simulink model "PlantaPIL"  (R2022b)
settings: Solver=ode1  StartTime=0.0  StopTime=SIMULPARAM.T_end  FixedStep=SIMULPARAM.Ts  RelTol=1e-3  EnableMultiTasking=on
InitFcn:
  | System_Parameters;
StopFcn:
  | ShowResults;
undefined symbols (not defined in the file or in its folder): Bat_cell, C_fil, C_fil_0, ENV, IPM, Ki_current_bat, Ki_current_sc, Ki_d_cur, Ki_q_cur, Kp_current_bat, Kp_current_sc, Kp_d_cur, Kp_q_cur, Kp_voltage, Kp_Vveh, L_bat, L_sc, n_bat_par, n_bat_seri, n_sc_par, n_sc_seri, Nbat, Ninv, Nsc, P1_I, P_I, R1_on, R_on, Rth, SC_modul, SC_pack, u_dc_ref, VEH
libraries: esp32_device_config_lib x1, simulink x1
(part 1 of 2)
settings Model: DataDictionary=MySharedDict.sldd  SILPILSystemUnderTest=refmodels  CodeVerificationMode=processor-in-the-loop (pil)  Creator=coins  LastModifiedBy=crist
settings SolverCC: AlgebraicLoopSolver=LineSearch  PositivePriorityOrder=on  AutoInsertRateTranBlk=on
settings DataIOCC: SignalLogging=off
settings OptimizationCC: EnhancedBackFolding=on  PassReuseOutputArgsAs=Individual arguments  ZeroExternalMemoryAtStartup=off  ZeroInternalMemoryAtStartup=off  OptimizeBlockOrder=speed  DifferentSizesBufferReuse=on  OptimizationCustomize=off  EfficientTunableParamExpr=on
settings DebuggingCC: ParameterTunabilityLossMsg=error  UnconnectedInputMsg=warning  UnconnectedOutputMsg=warning  UnconnectedLineMsg=warning  ModelReferenceSymbolNameMessage=none  PregeneratedLibrarySubsystemCodeDiagnostic=none  SFMachineParentedDataDiag=warning  ArithmeticOperatorsInVariantConditions=warning
settings HardwareCC: ProdBitPerPointer=32  ProdBitPerSizeT=32  ProdBitPerPtrDiffT=32  ProdLargestAtomicInteger=Long  ProdLargestAtomicFloat=Double  ProdWordSize=32  ProdHWDeviceType=Cadence Design Systems (Tensilica)->Espressif Xtensa single-/dual-core 32-bit LX6 microprocessor
settings ModelReferenceCC: UpdateModelReferenceTargets=Force  EnableRefExpFcnMdlSchedulingChecks=on
settings SFSimCC: MATLABDynamicMemAlloc=off  CustomCodeUndefinedFunction=UseInterfaceOnly
settings RTWCC: Description=Waijung 2 ESP32 target  SystemTargetFile=esp32.tlc  TemplateMakefile=esp32.tmf  RetainRTWFile=on  CreateSILPILBlock=PIL  CodeExecutionProfiling=on  DLArmComputeVersion=19.05
settings CodeAppCC: ForceParamTrailComments=on  IgnoreCustomStorageClasses=off  OperatorAnnotations=on  SimulinkDataObjDesc=on  SFDataObjDesc=on  InsertBlockDesc=on
settings STFCustomTargetCC: TargetLangStandard=C99 (ISO)  MultiwordLength=256  ModelReferenceCompliant=off  CombineOutputUpdateFcns=on  ERTCustomFileBanners=on  SupportContinuousTime=off  SupportNonInlinedSFcns=off  RemoveResetFunc=on  MATLABClassNameForMDSCustomization=Simulink.SoftwareTarget.ERTCustomization  SystemTargetFile=esp32.tlc
settings ERTTargetCC: TargetLangStandard=C99 (ISO)  ModelReferenceCompliant=off  ParMdlRefBuildCompliant=off  CompOptLevelCompliant=off  ConcurrentExecutionCompliant=off  ModelStepFunctionPrototypeControlCompliant=off  CPPClassGenCompliant=off  UseToolchainInfoCompliant=off  ExtModeStaticAlloc=on  ExtModeStaticAllocSize=2048  ERTSrcFileBannerTemplate=esp32_code_template.cgt  ERTHdrFileBannerTemplate=esp32_code_template.cgt  ERTDataSrcFileTemplate=esp32_code_template.cgt  ERTDataHdrFileTemplate=esp32_code_template.cgt  ERTCustomFileTemplate=esp32_file_process.tlc

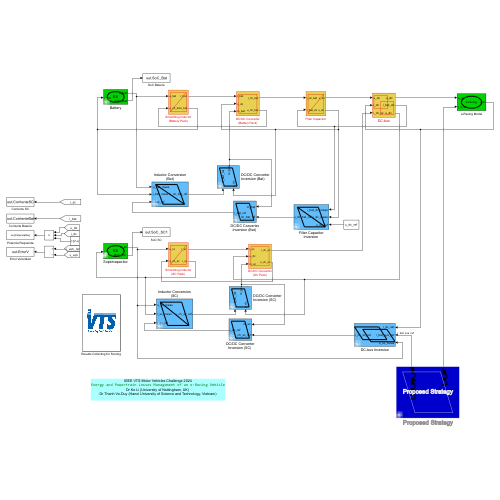
[thumbnail: Simulink's stored preview of the top-level diagram]
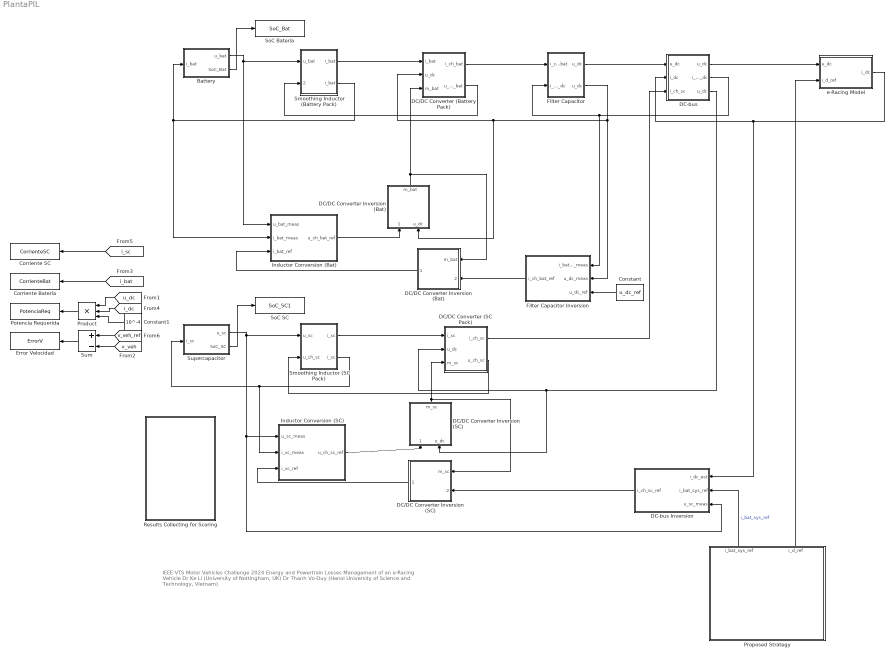
== system PlantaPIL ==
  note: IEEE VTS Motor Vehicles Challenge 2024
      | Energy and Powertrain Losses Management of an e-Racing Vehicle
      | Dr Ke Li (University of Nottingham, UK)
      | Dr Thanh Vo-Duy (Hanoi University of Science and Technology, Vietnam)
  Battery : Subsystem  AncestorBlock=simulink/REM/SE
      mask Display:
      | plot(0,0,100,100, 1.2*[50,57.68,60.77,63.08,64.97,66.58,68,69.26,70.4, 	71.42,72.36,78.28,80,78.28,72.36,71.42,70.4, 	69.26,68,66.58,64.97,63.08,60.77,57.68,50,42.32, 	39.23,36.92,35.03,33.42,32,30.74,29.6,28.58, 	27.64,21.72,20,21.72,27.64,28.58,29.6,30.74,32, 	33.42,35.03,36.92,39.23,42.32,50]-10, 1.2*[20,21,22,23,24,25,26,27,28,29,30,40,50,60,70,71,72, 	73,74,75,76,77,78,79,80,79,78,77,76,75,74,73,72, 	71,70,60,50,40,30,29,28,27,26,25,24,23,22,21,20]-10)
      | disp('ES')
  Constant : Constant  Value=u_dc_ref
  Constant1 : Constant  Value=10^-4
  Corriente Batería : ToWorkspace  VariableName=CorrienteBat  SaveFormat=Structure With Time  SampleTime=-1
  Corriente SC : ToWorkspace  VariableName=CorrienteSC  SaveFormat=Structure With Time  SampleTime=-1
  DC-bus : Subsystem  mask(CM){}
      mask Display: plot(0,0,100,100,[35,35,95,95,35],[65,10,10,65,65], [5,5,65,65,5],[90,35,35,90,90])
  DC-bus Inversion : Subsystem  AncestorBlock=simulink/SMC/Bloc de pondération
      mask Display: plot(0,0,100,100,[20,40,100,80,20],[75,20,20,75,75], [0,20,80,60,0],[85,30,30,85,85])
  DC/DC Converter (Battery Pack) : Subsystem
      mask Display: plot(0,0,100,100,[10,10,90,90,10],[90,10,10,90,90])
  DC/DC Converter (SC Pack) : Subsystem
      mask Display: plot(0,0,100,100,[10,10,90,90,10],[90,10,10,90,90])
  "DC/DC Converter Inversion (Bat) " : Subsystem  AncestorBlock=simulink/SMC/Inversion EC avec mesure
      mask Display: plot(0,0,100,100,[10,30,90,70,10],[90,10,10,90,90])
  "DC/DC Converter Inversion (Bat)  " : Subsystem  AncestorBlock=simulink/SMC/Inversion EC avec mesure
      mask Display: plot(0,0,100,100,[10,30,90,70,10],[90,10,10,90,90])
  DC/DC Converter Inversion (SC) : Subsystem  AncestorBlock=simulink/SMC/Inversion EC avec mesure
      mask Display: plot(0,0,100,100,[10,30,90,70,10],[90,10,10,90,90])
  "DC/DC Converter Inversion (SC) " : Subsystem  AncestorBlock=simulink/SMC/Inversion EC avec mesure
      mask Display: plot(0,0,100,100,[10,30,90,70,10],[90,10,10,90,90])
  Error Velocidad : ToWorkspace  VariableName=ErrorV  SaveFormat=Structure With Time  SampleTime=-1
  Filter Capacitor : Subsystem  mask(CM){}
      mask Display: plot(0,0,100,100,[10,10,90,90,10],[90,10,10,90,90], [10,90],[10,90])
  "Filter Capacitor Inversion " : Subsystem  AncestorBlock=simulink/SMC/Asservissement Correcteur IP
      mask Display: plot(0,0,100,100, [10,30,90,70,10,90],[90,10,10,90,90,10])
  Inductor Conversion (Bat) : Subsystem  AncestorBlock=simulink/SMC/Asservissement Correcteur IP
      mask Display: plot(0,0,100,100, [10,30,90,70,10,90],[90,10,10,90,90,10])
  Inductor Conversion (SC) : Subsystem  AncestorBlock=simulink/SMC/Asservissement Correcteur IP
      mask Display: plot(0,0,100,100, [10,30,90,70,10,90],[90,10,10,90,90,10])
  Potencia Requerida : ToWorkspace  VariableName=PotenciaReq  SaveFormat=Structure With Time  SampleTime=-1
  Product : Product  Inputs=3
  Proposed Strategy : Subsystem  AncestorBlock=simulink/SMC/Inversion EC avec mesure
      mask Display:
      | disp('Proposed Strategy')
      | plot(0,0,100,100,[10,30,90,70,10],[90,10,10,90,90])
  Results Collecting for Scoring : Subsystem
      mask Display: image('VTS.png');
  Smoothing Inductor (Battery Pack) : Subsystem  mask(CM){}
      mask Display: plot(0,0,100,100,[10,10,90,90,10],[90,10,10,90,90], [10,90],[10,90])
  Smoothing Inductor (SC Pack) : Subsystem  mask(CM){}
      mask Display: plot(0,0,100,100,[10,10,90,90,10],[90,10,10,90,90], [10,90],[10,90])
  SoC Batería : ToWorkspace  VariableName=SoC_Bat  SaveFormat=Structure With Time  SampleTime=-1
  SoC SC : ToWorkspace  VariableName=SoC_SC1  SaveFormat=Structure With Time  SampleTime=-1
  Sum : Sum  Inputs=+-
  Supercapacitor : Subsystem  AncestorBlock=simulink/REM/SE
      mask Display:
      | plot(0,0,100,100, 1.2*[50,57.68,60.77,63.08,64.97,66.58,68,69.26,70.4, 	71.42,72.36,78.28,80,78.28,72.36,71.42,70.4, 	69.26,68,66.58,64.97,63.08,60.77,57.68,50,42.32, 	39.23,36.92,35.03,33.42,32,30.74,29.6,28.58, 	27.64,21.72,20,21.72,27.64,28.58,29.6,30.74,32, 	33.42,35.03,36.92,39.23,42.32,50]-10, 1.2*[20,21,22,23,24,25,26,27,28,29,30,40,50,60,70,71,72, 	73,74,75,76,77,78,79,80,79,78,77,76,75,74,73,72, 	71,70,60,50,40,30,29,28,27,26,25,24,23,22,21,20]-10)
      | disp('ES')
  e-Racing Model : Subsystem
      mask Display:
      | plot(0,0,100,100, 1.2*[50,57.68,60.77,63.08,64.97,66.58,68,69.26,70.4, 	71.42,72.36,78.28,80,78.28,72.36,71.42,70.4, 	69.26,68,66.58,64.97,63.08,60.77,57.68,50,42.32, 	39.23,36.92,35.03,33.42,32,30.74,29.6,28.58, 	27.64,21.72,20,21.72,27.64,28.58,29.6,30.74,32, 	33.42,35.03,36.92,39.23,42.32,50]-10, 1.2*[20,21,22,23,24,25,26,27,28,29,30,40,50,60,70,71,72, 	73,74,75,76,77,78,79,80,79,78,77,76,75,74,73,72, 	71,70,60,50,40,30,29,28,27,26,25,24,23,22,21,20]-10)
      | disp('e-racing')
  wires:
  Supercapacitor/1(u_sc) -> DC-bus Inversion/3(u_sc_meas), Inductor Conversion (SC)/1(u_sc_meas), Smoothing Inductor (SC Pack)/1(u_sc)
  Smoothing Inductor (SC Pack)/2(i_sc) -> Supercapacitor/1(i_sc), Inductor Conversion (SC)/2(i_sc_meas)
  Smoothing Inductor (SC Pack)/1("i_sc ") -> DC/DC Converter (SC Pack)/1(i_sc)
  DC/DC Converter (SC Pack)/2(u_ch_sc) -> Smoothing Inductor (SC Pack)/2(u_ch_sc)
  DC-bus/1("u_dc  ") -> e-Racing Model/1(u_dc)
  DC/DC Converter (SC Pack)/1(i_ch_sc) -> DC-bus/3(i_ch_sc)
  DC-bus/3("u_dc   ") -> DC/DC Converter Inversion (SC)/2(u_dc), DC/DC Converter (SC Pack)/2(u_dc)
  Battery/1(u_bat) -> Inductor Conversion (Bat)/1(u_bat_meas), Smoothing Inductor (Battery Pack)/1(u_bat)
  Smoothing Inductor (Battery Pack)/2(i_bat) -> Inductor Conversion (Bat)/2(i_bat_meas), Battery/1(i_bat)
  Filter Capacitor/2("u_dc ") -> DC/DC Converter (Battery Pack)/2(u_dc), "DC/DC Converter Inversion (Bat)  "/2(u_dc), "Filter Capacitor Inversion "/2(u_dc_meas)
  Constant/1 -> "Filter Capacitor Inversion "/3(u_dc_ref)
  "DC/DC Converter Inversion (Bat)  "/1(m_bat) -> DC/DC Converter (Battery Pack)/3(m_bat), "DC/DC Converter Inversion (Bat) "/1(m_bat)
  "DC/DC Converter Inversion (SC) "/1(i_sc_ref) -> Inductor Conversion (SC)/3(i_sc_ref)
  Inductor Conversion (SC)/1(u_ch_sc_ref) -> DC/DC Converter Inversion (SC)/1(u_ch_sc_ref)
  DC/DC Converter Inversion (SC)/1(m_sc) -> DC/DC Converter (SC Pack)/3(m_sc), "DC/DC Converter Inversion (SC) "/1(m_sc)
  "Filter Capacitor Inversion "/1(i_ch_bat_ref) -> "DC/DC Converter Inversion (Bat) "/2(i_ch_bat_ref)
  "DC/DC Converter Inversion (Bat) "/1(i_bat_ref) -> Inductor Conversion (Bat)/3(i_bat_ref)
  Inductor Conversion (Bat)/1(u_ch_bat_ref) -> "DC/DC Converter Inversion (Bat)  "/1(u_ch_bat_ref)
  DC/DC Converter (Battery Pack)/2(u_ch_bat) -> Smoothing Inductor (Battery Pack)/2(u_ch_bat)
  DC/DC Converter (Battery Pack)/1(i_ch_bat) -> Filter Capacitor/1(i_ch_bat)
  Smoothing Inductor (Battery Pack)/1("i_bat ") -> DC/DC Converter (Battery Pack)/1(i_bat)
  e-Racing Model/1(i_dc) -> DC-bus Inversion/1(i_dc_est), DC-bus/2(i_dc)
  Filter Capacitor/1(u_dc) -> DC-bus/1(u_dc)
  DC-bus Inversion/1(i_ch_sc_ref) -> "DC/DC Converter Inversion (SC) "/2(i_ch_sc_ref)
  Proposed Strategy/1(i_bat_sys_ref) -> DC-bus Inversion/2(i_bat_sys_ref)  "i_bat_sys_ref"
  DC-bus/2(i_bat_dc) -> "Filter Capacitor Inversion "/1(i_bat_dc_meas), Filter Capacitor/2(i_bat_dc)
  Proposed Strategy/2("i_d_ref ") -> e-Racing Model/2(i_d_ref)
  Supercapacitor/2("SoC_SC ") -> SoC SC/1
  Battery/2(SoC_Bat) -> SoC Batería/1
  [i_sc] -> Corriente SC/1
  [i_bat] -> Corriente Batería/1
  Constant1/1 -> Product/3
  Product/1 -> Potencia Requerida/1
  [i_dc] -> Product/2
  [u_dc] -> Product/1
  [v_veh] -> Sum/2
  [v_veh_ref] -> Sum/1
  Sum/1 -> Error Velocidad/1

== system PlantaPIL/Battery ==
  i_bat : Inport
  Constant : Constant
  Gain : Gain  Gain=1/(3600*Bat_cell.Capacity)
  Gain1 : Gain  Gain=1/n_bat_par
  Gain2 : Gain  Gain=Bat_cell.InternalRes
  Gain3 : Gain  Gain=n_bat_seri
  Gain4 : Gain  Gain=100
  Gain5 : Gain  Gain=-1
  Integrator : Integrator  InitialCondition=1
  OCV(SoC) : Lookup_n-D  NumberOfTableDimensions=1  BreakpointsForDimension1=Bat_cell.SoC  Table=Bat_cell.OCV  InternalRulePriority=Speed  RndMeth=Simplest
  Subtract : Sum  Inputs=+-
  Subtract1 : Sum  Inputs=+-
  u_bat : Outport  InitialOutput=0  VectorParamsAs1DForOutWhenUnconnected=off
  SoC_Bat : Outport  Port=2  InitialOutput=0  VectorParamsAs1DForOutWhenUnconnected=off
  tag scope: Bat_soc=global, i_bat=global, i_bat_cell=global, u_bat=global, u_bat_cell=global
  wires:
  Gain/1 -> Integrator/1
  i_bat/1 -> [i_bat], Gain1/1
  Gain1/1 -> Gain2/1, Gain5/1, [i_bat_cell]  "i_bat_cell"
  OCV(SoC)/1 -> Subtract1/1  "OCV"
  Gain2/1 -> Subtract1/2
  Subtract1/1 -> [u_bat_cell], Gain3/1  "u_bat_cell"
  Gain3/1 -> [u_bat], u_bat/1
  Constant/1 -> Subtract/1
  Integrator/1 -> Gain4/1, Subtract/2
  Gain4/1 -> SoC_Bat/1, [Bat_soc]  "Battery's SoC"
  Subtract/1 -> OCV(SoC)/1
  Gain5/1 -> Gain/1

== system PlantaPIL/DC-bus ==
  u_dc : Inport
  i_dc : Inport  Port=2
  i_ch_sc : Inport  Port=3
  For scoring : ToWorkspace  VariableName=i_dc_meas  SampleTime=-1
      settings: Decimation=SIMULPARAM.Decimation
  Subtract : Sum  Inputs=+-
  "u_dc  " : Outport  InitialOutput=0  VectorParamsAs1DForOutWhenUnconnected=off
  i_bat_dc : Outport  Port=2  InitialOutput=0  VectorParamsAs1DForOutWhenUnconnected=off
  "u_dc   " : Outport  Port=3  InitialOutput=0  VectorParamsAs1DForOutWhenUnconnected=off
  wires:
  u_dc/1 -> "u_dc   "/1, "u_dc  "/1
  i_dc/1 -> For scoring/1, Subtract/1
  Subtract/1 -> i_bat_dc/1
  i_ch_sc/1 -> Subtract/2

== system PlantaPIL/DC-bus Inversion ==
  i_dc_est : Inport
  i_bat_sys_ref : Inport  Port=2
  u_sc_meas : Inport  Port=3
  SC Limitation : Subsystem
  Subtract1 : Sum  Inputs=+-
  i_ch_sc_ref : Outport  InitialOutput=0  VectorParamsAs1DForOutWhenUnconnected=off
  tag scope: i_ch_sc_ref=global
  wires:
  SC Limitation/1(i_bat_ref) -> Subtract1/2
  u_sc_meas/1 -> SC Limitation/2(u_sc_meas)
  i_bat_sys_ref/1 -> SC Limitation/3(i_bat_ref_cal)
  i_dc_est/1 -> Subtract1/1, SC Limitation/1(i_dc)
  Subtract1/1 -> [i_ch_sc_ref], i_ch_sc_ref/1

== system PlantaPIL/DC//DC Converter (Battery Pack) ==
  i_bat : Inport
  u_dc : Inport  Port=2
  m_bat : Inport  Port=3
  Converter loss : Subsystem
  Divide : Product  Inputs=*/
  Product{,1..3} (4 alike) : Product
  Saturation : Saturate  UpperLimit=1  LowerLimit=0
  Switch : Switch  Criteria=u2 > Threshold  SaturateOnIntegerOverflow=off  InputSameDT=off
  i_ch_bat : Outport  InitialOutput=0  VectorParamsAs1DForOutWhenUnconnected=off
  u_ch_bat : Outport  Port=2  InitialOutput=0  VectorParamsAs1DForOutWhenUnconnected=off
  tag scope: Ploss_bat=global, Ts1_bat=global, Ts2_bat=global
  wires:
  Product/1 -> i_ch_bat/1
  i_bat/1 -> Converter loss/1(i_bat), Divide/1, Product3/2, Product1/1
  Product3/1 -> Switch/1
  Product1/1 -> Switch/2
  Switch/1 -> Product/1
  u_dc/1 -> Converter loss/2(u_dc), Product2/1
  Product2/1 -> u_ch_bat/1, Product1/2
  Divide/1 -> Switch/3
  m_bat/1 -> Converter loss/3(m_bat), Saturation/1
  Saturation/1 -> Product/2, Product2/2
  Converter loss/1(eff) -> Divide/2, Product3/1
  Converter loss/2(T_S1) -> [Ts1_bat]
  Converter loss/3(T_S2) -> [Ts2_bat]
  Converter loss/4(Ploss) -> [Ploss_bat]

== system PlantaPIL/DC//DC Converter (SC Pack) ==
  i_sc : Inport
  u_dc : Inport  Port=2
  m_sc : Inport  Port=3
  Converter loss : Subsystem
  Divide : Product  Inputs=*/
  Product{,1..3} (4 alike) : Product
  Saturation : Saturate  UpperLimit=1  LowerLimit=0
  Switch : Switch  Criteria=u2 > Threshold  SaturateOnIntegerOverflow=off  InputSameDT=off
  i_ch_sc : Outport  InitialOutput=0  VectorParamsAs1DForOutWhenUnconnected=off
  u_ch_sc : Outport  Port=2  InitialOutput=0  VectorParamsAs1DForOutWhenUnconnected=off
  tag scope: Ploss_sc=global, Ts1_sc=global, Ts2_sc=global, i_ch_sc=global
  wires:
  Product2/1 -> u_ch_sc/1, Product1/2
  m_sc/1 -> Converter loss/3(m_sc), Saturation/1
  u_dc/1 -> Converter loss/2(u_dc), Product2/1
  Product/1 -> [i_ch_sc], i_ch_sc/1
  Switch/1 -> Product/1
  Product3/1 -> Switch/1
  Divide/1 -> Switch/3
  Product1/1 -> Switch/2
  i_sc/1 -> Converter loss/1(i_sc), Product3/1, Divide/1, Product1/1
  Saturation/1 -> Product2/2, Product/2
  Converter loss/1(eff) -> Product3/2, Divide/2
  Converter loss/2(T_S1) -> [Ts1_sc]
  Converter loss/3(T_S2) -> [Ts2_sc]
  Converter loss/4(Ploss) -> [Ploss_sc]

== system PlantaPIL/DC//DC Converter Inversion (Bat)  ==
  m_bat : Inport
  i_ch_bat_ref : Inport  Port=2
  Divide : Product  Inputs=*/
  Memory : Memory  InitialCondition=0.1
  i_bat_ref : Outport  InitialOutput=0  VectorParamsAs1DForOutWhenUnconnected=off
  tag scope: i_bat_ref=global
  wires:
  Divide/1 -> [i_bat_ref], i_bat_ref/1
  i_ch_bat_ref/1 -> Divide/1
  Memory/1 -> Divide/2
  m_bat/1 -> Memory/1

== system PlantaPIL/DC//DC Converter Inversion (Bat)   ==
  u_ch_bat_ref : Inport
  u_dc : Inport  Port=2
  Divide : Product  Inputs=*/
  Saturation1 : Saturate  UpperLimit=1  LowerLimit=0.00001
  m_bat : Outport  InitialOutput=0  VectorParamsAs1DForOutWhenUnconnected=off
  tag scope: m_bat=global
  wires:
  u_ch_bat_ref/1 -> Divide/1
  u_dc/1 -> Divide/2
  Divide/1 -> Saturation1/1
  Saturation1/1 -> [m_bat], m_bat/1

== system PlantaPIL/DC//DC Converter Inversion (SC) ==
  u_ch_sc_ref : Inport
  u_dc : Inport  Port=2
  Divide : Product  Inputs=*/
  Saturation1 : Saturate  UpperLimit=1  LowerLimit=0.00001
  m_sc : Outport  InitialOutput=0  VectorParamsAs1DForOutWhenUnconnected=off
  tag scope: m_sc=global
  wires:
  u_ch_sc_ref/1 -> Divide/1
  u_dc/1 -> Divide/2
  Divide/1 -> Saturation1/1
  Saturation1/1 -> [m_sc], m_sc/1

== system PlantaPIL/DC//DC Converter Inversion (SC)  ==
  m_sc : Inport
  i_ch_sc_ref : Inport  Port=2
  Divide : Product  Inputs=*/
  Memory : Memory  InitialCondition=0.1
  i_sc_ref : Outport  InitialOutput=0  VectorParamsAs1DForOutWhenUnconnected=off
  tag scope: i_sc_ref=global
  wires:
  Divide/1 -> [i_sc_ref], i_sc_ref/1
  i_ch_sc_ref/1 -> Divide/1
  Memory/1 -> Divide/2
  m_sc/1 -> Memory/1

== system PlantaPIL/Filter Capacitor ==
  i_ch_bat : Inport
  i_bat_dc : Inport  Port=2
  Gain : Gain  Gain=1/C_fil
  Integrator : Integrator  InitialCondition=C_fil_0
  Sum : Sum  Inputs=|+-
  u_dc : Outport  InitialOutput=0  VectorParamsAs1DForOutWhenUnconnected=off
  "u_dc " : Outport  Port=2  InitialOutput=0  VectorParamsAs1DForOutWhenUnconnected=off
  tag scope: i_bat_dc=global, u_dc=global
  wires:
  i_ch_bat/1 -> Sum/1
  i_bat_dc/1 -> [i_bat_dc], Sum/2
  Gain/1 -> Integrator/1
  Sum/1 -> Gain/1
  Integrator/1 -> "u_dc "/1, [u_dc], u_dc/1

== system PlantaPIL/Filter Capacitor Inversion  ==
  i_bat_dc_meas : Inport
  u_dc_meas : Inport  Port=2
  u_dc_ref : Inport  Port=3
  Add : Sum
  Gain : Gain  Gain=Kp_voltage
  Subtract : Sum  Inputs=-+
  i_ch_bat_ref : Outport  InitialOutput=0  VectorParamsAs1DForOutWhenUnconnected=off
  tag scope: i_ch_bat_ref=global
  wires:
  u_dc_ref/1 -> Subtract/2
  u_dc_meas/1 -> Subtract/1
  Subtract/1 -> Gain/1
  i_bat_dc_meas/1 -> Add/1
  Gain/1 -> Add/2
  Add/1 -> [i_ch_bat_ref], i_ch_bat_ref/1

== system PlantaPIL/Inductor Conversion (Bat) ==
  u_bat_meas : Inport
  i_bat_meas : Inport  Port=2
  i_bat_ref : Inport  Port=3
  Add : Sum  Inputs=+-
  Gain : Gain  Gain=Kp_current_bat
  Gain1 : Gain  Gain=Ki_current_bat
  Integrator : Integrator
  Subtract : Sum  Inputs=-+
  Sum : Sum  Inputs=|++
  u_ch_bat_ref : Outport  InitialOutput=0  VectorParamsAs1DForOutWhenUnconnected=off
  tag scope: u_ch_bat_ref=global
  wires:
  Add/1 -> [u_ch_bat_ref], u_ch_bat_ref/1
  u_bat_meas/1 -> Add/1
  Subtract/1 -> Gain/1, Gain1/1
  i_bat_meas/1 -> Subtract/1
  i_bat_ref/1 -> Subtract/2
  Gain1/1 -> Integrator/1
  Gain/1 -> Sum/2
  Sum/1 -> Add/2
  Integrator/1 -> Sum/1

== system PlantaPIL/Inductor Conversion (SC) ==
  u_sc_meas : Inport
  i_sc_meas : Inport  Port=2
  i_sc_ref : Inport  Port=3
  Add : Sum  Inputs=+-
  Gain : Gain  Gain=Kp_current_sc
  Gain1 : Gain  Gain=Ki_current_sc
  Integrator : Integrator
  Subtract : Sum  Inputs=-+
  Sum : Sum  Inputs=|++
  u_ch_sc_ref : Outport  InitialOutput=0  VectorParamsAs1DForOutWhenUnconnected=off
  tag scope: u_ch_sc_ref=global
  wires:
  Integrator/1 -> Sum/1
  Sum/1 -> Add/2
  Gain/1 -> Sum/2
  Gain1/1 -> Integrator/1
  i_sc_ref/1 -> Subtract/2
  i_sc_meas/1 -> Subtract/1
  Subtract/1 -> Gain/1, Gain1/1
  u_sc_meas/1 -> Add/1
  Add/1 -> [u_ch_sc_ref], u_ch_sc_ref/1

== system PlantaPIL/Proposed Strategy ==
  note: Implementación Embebida de una Estrategia de Control y Gestión
      | de Energía para un Vehículo Eléctrico con Batería y
      | Supercapacitor
  note: Estrategia de gestion de energías
  note: Cristhian José Narváez Gallon
      | Juan Manuel Rodriguez Montoya
      | José Reinaldo Vuelvas Quintana
      | Juan Diego Valladolid
  Controlador : ModelReference  ModelNameDialog=ControladorEmbebido.slx  SimulationMode=Processor-in-the-loop (PIL)  ModelReferenceVersion=7.24
  Processor-in-the-loop Host Setup : esp32_device_config_lib/Processor-in-the-loop Host Setup  blockid=ProposedStrategyProcessorintheloopHostSetup
      settings: SourceProductName=Waijung 2 Blockset
  Saturation : Saturate  UpperLimit=150  LowerLimit=0
  Saturation1 : Saturate  UpperLimit=0  LowerLimit=-100
  Scope : Scope
  Scope1 : Scope
  Variables controlador : Subsystem
  i_bat_sys_ref : Outport  InitialOutput=0  VectorParamsAs1DForOutWhenUnconnected=off
  "i_d_ref " : Outport  Port=2  InitialOutput=0  VectorParamsAs1DForOutWhenUnconnected=off
  wires:
  Saturation/1 -> i_bat_sys_ref/1, Scope/1
  Saturation1/1 -> "i_d_ref "/1, Scope1/1
  Variables controlador/1(SoC_Bat) -> Controlador/1
  Variables controlador/2(SoC_SC) -> Controlador/2
  Variables controlador/3(Potencia_Req) -> Controlador/3
  Variables controlador/4(Velocidad_w) -> Controlador/4
  Variables controlador/5(ErrorVelocidad) -> Controlador/5
  Controlador/2 -> Saturation1/1
  Controlador/1 -> Saturation/1

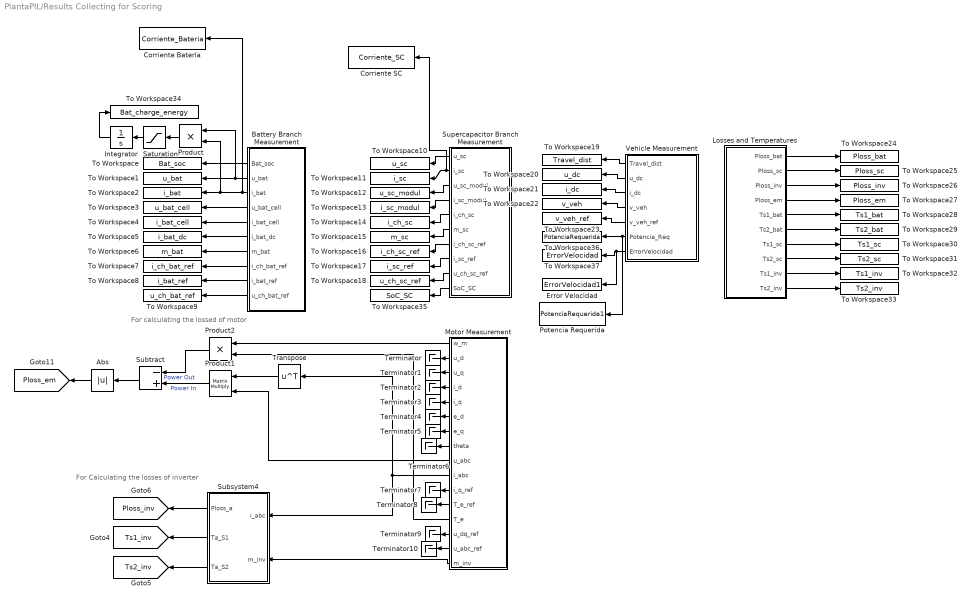
== system PlantaPIL/Results Collecting for Scoring ==
  note: For Calculating the losses of inverter
  note: For calculating the lossed of motor
  Abs : Abs  SaturateOnIntegerOverflow=off
  Battery Branch Measurement : Subsystem
  Corriente Batería : ToWorkspace  VariableName=Corriente_Bateria  SaveFormat=Structure With Time  SampleTime=-1
  Corriente SC : ToWorkspace  VariableName=Corriente_SC  SaveFormat=Structure With Time  SampleTime=-1
  Error Velocidad : ToWorkspace  VariableName=ErrorVelocidad1  SaveFormat=Structure With Time  SampleTime=-1
      settings: Decimation=SIMULPARAM.Decimation
  Integrator : Integrator
  Losses and Temperatures : Subsystem
  Motor Measurement : Subsystem
  Potencia Requerida : ToWorkspace  VariableName=PotenciaRequerida1  SaveFormat=Structure With Time  SampleTime=-1
  Product : Product
  Product1 : Product  Multiplication=Matrix(*)
  Product2 : Product
  Saturation : Saturate  UpperLimit=0  LowerLimit=-inf
  Subsystem4 : Subsystem
  Subtract : Sum  Inputs=-+
  Supercapacitor Branch Measurement : Subsystem
  Terminator{,1..10} (11 alike) : Terminator
  To Workspace : ToWorkspace  VariableName=Bat_soc  SampleTime=-1
      settings: Decimation=SIMULPARAM.Decimation
  To Workspace1 : ToWorkspace  VariableName=u_bat  SampleTime=-1
      settings: Decimation=SIMULPARAM.Decimation
  To Workspace10 : ToWorkspace  VariableName=u_sc  SampleTime=-1
      settings: Decimation=SIMULPARAM.Decimation
  To Workspace11 : ToWorkspace  VariableName=i_sc  SampleTime=-1
      settings: Decimation=SIMULPARAM.Decimation
  To Workspace12 : ToWorkspace  VariableName=u_sc_modul  SampleTime=-1
      settings: Decimation=SIMULPARAM.Decimation
  To Workspace13 : ToWorkspace  VariableName=i_sc_modul  SampleTime=-1
      settings: Decimation=SIMULPARAM.Decimation
  To Workspace14 : ToWorkspace  VariableName=i_ch_sc  SampleTime=-1
      settings: Decimation=SIMULPARAM.Decimation
  To Workspace15 : ToWorkspace  VariableName=m_sc  SampleTime=-1
      settings: Decimation=SIMULPARAM.Decimation
  To Workspace16 : ToWorkspace  VariableName=i_ch_sc_ref  SampleTime=-1
      settings: Decimation=SIMULPARAM.Decimation
  To Workspace17 : ToWorkspace  VariableName=i_sc_ref  SampleTime=-1
      settings: Decimation=SIMULPARAM.Decimation
  To Workspace18 : ToWorkspace  VariableName=u_ch_sc_ref  SampleTime=-1
      settings: Decimation=SIMULPARAM.Decimation
  To Workspace19 : ToWorkspace  VariableName=Travel_dist  SampleTime=-1
      settings: Decimation=SIMULPARAM.Decimation
  To Workspace2 : ToWorkspace  VariableName=i_bat  SampleTime=-1
      settings: Decimation=SIMULPARAM.Decimation
  To Workspace20 : ToWorkspace  VariableName=u_dc  SampleTime=-1
      settings: Decimation=SIMULPARAM.Decimation
  To Workspace21 : ToWorkspace  VariableName=i_dc  SampleTime=-1
      settings: Decimation=SIMULPARAM.Decimation
  To Workspace22 : ToWorkspace  VariableName=v_veh  SampleTime=-1
      settings: Decimation=SIMULPARAM.Decimation
  To Workspace23 : ToWorkspace  VariableName=v_veh_ref  SampleTime=-1
      settings: Decimation=SIMULPARAM.Decimation
  To Workspace24 : ToWorkspace  VariableName=Ploss_bat  SampleTime=-1
      settings: Decimation=SIMULPARAM.Decimation
  To Workspace25 : ToWorkspace  VariableName=Ploss_sc  SampleTime=-1
      settings: Decimation=SIMULPARAM.Decimation
  To Workspace26 : ToWorkspace  VariableName=Ploss_inv  SampleTime=-1
      settings: Decimation=SIMULPARAM.Decimation
  To Workspace27 : ToWorkspace  VariableName=Ploss_em  SampleTime=-1
      settings: Decimation=SIMULPARAM.Decimation
  To Workspace28 : ToWorkspace  VariableName=Ts1_bat  SampleTime=-1
      settings: Decimation=SIMULPARAM.Decimation
  To Workspace29 : ToWorkspace  VariableName=Ts2_bat  SampleTime=-1
      settings: Decimation=SIMULPARAM.Decimation
  To Workspace3 : ToWorkspace  VariableName=u_bat_cell  SampleTime=-1
      settings: Decimation=SIMULPARAM.Decimation
  To Workspace30 : ToWorkspace  VariableName=Ts1_sc  SampleTime=-1
      settings: Decimation=SIMULPARAM.Decimation
  To Workspace31 : ToWorkspace  VariableName=Ts2_sc  SampleTime=-1
      settings: Decimation=SIMULPARAM.Decimation
  To Workspace32 : ToWorkspace  VariableName=Ts1_inv  SampleTime=-1
      settings: Decimation=SIMULPARAM.Decimation
  To Workspace33 : ToWorkspace  VariableName=Ts2_inv  SampleTime=-1
      settings: Decimation=SIMULPARAM.Decimation
  To Workspace34 : ToWorkspace  VariableName=Bat_charge_energy  SampleTime=-1
      settings: Decimation=SIMULPARAM.Decimation
  To Workspace35 : ToWorkspace  VariableName=SoC_SC  SampleTime=-1
      settings: Decimation=SIMULPARAM.Decimation
  To Workspace36 : ToWorkspace  VariableName=PotenciaRequerida  SampleTime=-1
      settings: Decimation=SIMULPARAM.Decimation
  To Workspace37 : ToWorkspace  VariableName=ErrorVelocidad  SampleTime=-1
      settings: Decimation=SIMULPARAM.Decimation
  To Workspace4 : ToWorkspace  VariableName=i_bat_cell  SampleTime=-1
      settings: Decimation=SIMULPARAM.Decimation
  To Workspace5 : ToWorkspace  VariableName=i_bat_dc  SampleTime=-1
      settings: Decimation=SIMULPARAM.Decimation
  To Workspace6 : ToWorkspace  VariableName=m_bat  SampleTime=-1
      settings: Decimation=SIMULPARAM.Decimation
  To Workspace7 : ToWorkspace  VariableName=i_ch_bat_ref  SampleTime=-1
      settings: Decimation=SIMULPARAM.Decimation
  To Workspace8 : ToWorkspace  VariableName=i_bat_ref  SampleTime=-1
      settings: Decimation=SIMULPARAM.Decimation
  To Workspace9 : ToWorkspace  VariableName=u_ch_bat_ref  SampleTime=-1
      settings: Decimation=SIMULPARAM.Decimation
  Transpose : Math  Operator=transpose
  Vehicle Measurement : Subsystem
  tag scope: Ploss_em=global, Ploss_inv=global, Ts1_inv=global, Ts2_inv=global
  wires:
  Battery Branch Measurement/1(Bat_soc) -> To Workspace/1
  Battery Branch Measurement/2(u_bat) -> Product/1, To Workspace1/1
  Battery Branch Measurement/3(i_bat) -> Corriente Batería/1, Product/2, To Workspace2/1
  Battery Branch Measurement/4(u_bat_cell) -> To Workspace3/1
  Battery Branch Measurement/5(i_bat_cell) -> To Workspace4/1
  Battery Branch Measurement/6(i_bat_dc) -> To Workspace5/1
  Battery Branch Measurement/7(m_bat) -> To Workspace6/1
  Battery Branch Measurement/8(i_ch_bat_ref) -> To Workspace7/1
  Battery Branch Measurement/9(i_bat_ref) -> To Workspace8/1
  Battery Branch Measurement/10(u_ch_bat_ref) -> To Workspace9/1
  Supercapacitor Branch Measurement/1(u_sc) -> To Workspace10/1
  Supercapacitor Branch Measurement/2(i_sc) -> Corriente SC/1, To Workspace11/1
  Supercapacitor Branch Measurement/3(u_sc_modul) -> To Workspace12/1
  Supercapacitor Branch Measurement/4(i_sc_modul) -> To Workspace13/1
  Supercapacitor Branch Measurement/5(i_ch_sc) -> To Workspace14/1
  Supercapacitor Branch Measurement/6(m_sc) -> To Workspace15/1
  Supercapacitor Branch Measurement/7(i_ch_sc_ref) -> To Workspace16/1
  Supercapacitor Branch Measurement/8(i_sc_ref) -> To Workspace17/1
  Supercapacitor Branch Measurement/9(u_ch_sc_ref) -> To Workspace18/1
  Vehicle Measurement/1(Travel_dist) -> To Workspace19/1
  Vehicle Measurement/2(u_dc) -> To Workspace20/1
  Vehicle Measurement/3(i_dc) -> To Workspace21/1
  Vehicle Measurement/4(v_veh) -> To Workspace22/1
  Vehicle Measurement/5(v_veh_ref) -> To Workspace23/1
  Losses and Temperatures/1(Ploss_bat) -> To Workspace24/1
  Losses and Temperatures/2(Ploss_sc) -> To Workspace25/1
  Losses and Temperatures/3(Ploss_inv) -> To Workspace26/1
  Losses and Temperatures/4(Ploss_em) -> To Workspace27/1
  Losses and Temperatures/8(Ts2_sc) -> To Workspace31/1
  Losses and Temperatures/7(Ts1_sc) -> To Workspace30/1
  Losses and Temperatures/5(Ts1_bat) -> To Workspace28/1
  Losses and Temperatures/6(Ts2_bat) -> To Workspace29/1
  Losses and Temperatures/9(Ts1_inv) -> To Workspace32/1
  Losses and Temperatures/10(Ts2_inv) -> To Workspace33/1
  Saturation/1 -> Integrator/1
  Integrator/1 -> To Workspace34/1
  Product/1 -> Saturation/1
  Motor Measurement/1(w_m) -> Product2/1
  Product2/1 -> Subtract/1  "Power Out"
  Subsystem4/2(Ta_S1) -> [Ts1_inv]
  Abs/1 -> [Ploss_em]
  Transpose/1 -> Product1/1
  Motor Measurement/13(T_e) -> Product2/2
  Motor Measurement/9(u_abc) -> Product1/2
  Subsystem4/3(Ta_S2) -> [Ts2_inv]
  Subsystem4/1(Ploss_a) -> [Ploss_inv]
  Subtract/1 -> Abs/1
  Product1/1 -> Subtract/2  "Power In"
  Motor Measurement/10(i_abc) -> Transpose/1, Subsystem4/1(i_abc)
  Motor Measurement/16(m_inv) -> Subsystem4/2(m_inv)
  Motor Measurement/2(u_d) -> Terminator/1
  Motor Measurement/3(u_q) -> Terminator1/1
  Motor Measurement/4(i_d) -> Terminator2/1
  Motor Measurement/5(i_q) -> Terminator3/1
  Motor Measurement/6(e_d) -> Terminator4/1
  Motor Measurement/7(e_q) -> Terminator5/1
  Motor Measurement/11(i_q_ref) -> Terminator7/1
  Motor Measurement/12(T_e_ref) -> Terminator8/1
  Motor Measurement/15(u_abc_ref) -> Terminator10/1
  Motor Measurement/14(u_dq_ref) -> Terminator9/1
  Motor Measurement/8(theta) -> Terminator6/1
  Supercapacitor Branch Measurement/10(SoC_SC) -> To Workspace35/1
  Vehicle Measurement/6(Potencia_Req) -> Potencia Requerida/1, To Workspace36/1
  Vehicle Measurement/7(ErrorVelocidad) -> Error Velocidad/1, To Workspace37/1

== system PlantaPIL/Smoothing Inductor (Battery Pack) ==
  u_bat : Inport
  u_ch_bat : Inport  Port=2
  Sum : Sum  Inputs=|+-
  Transfer Fcn : TransferFcn  Denominator=[L_bat.L_sm L_bat.R_sm]
  "i_bat " : Outport  InitialOutput=0  VectorParamsAs1DForOutWhenUnconnected=off
  i_bat : Outport  Port=2  InitialOutput=0  VectorParamsAs1DForOutWhenUnconnected=off
  wires:
  Transfer Fcn/1 -> "i_bat "/1, i_bat/1
  Sum/1 -> Transfer Fcn/1
  u_ch_bat/1 -> Sum/2
  u_bat/1 -> Sum/1

== system PlantaPIL/Smoothing Inductor (SC Pack) ==
  u_sc : Inport
  u_ch_sc : Inport  Port=2
  Sum : Sum  Inputs=|+-
  Transfer Fcn : TransferFcn  Denominator=[L_sc.L_sm L_sc.R_sm]
  "i_sc " : Outport  InitialOutput=0  VectorParamsAs1DForOutWhenUnconnected=off
  i_sc : Outport  Port=2  InitialOutput=0  VectorParamsAs1DForOutWhenUnconnected=off
  wires:
  u_sc/1 -> Sum/1
  u_ch_sc/1 -> Sum/2
  Sum/1 -> Transfer Fcn/1
  Transfer Fcn/1 -> i_sc/1, "i_sc "/1

== system PlantaPIL/Supercapacitor ==
  i_sc : Inport
  Add : Sum  Inputs=+++
  Constant : Constant  Value=SC_modul.U_init
  Constant1 : Constant  Value=1/SC_modul.U_rated
  Constant2 : Constant  Value=10
  Gain : Gain  Gain=-1/SC_modul.C_rated
  Gain1 : Gain  Gain=n_sc_seri
  Gain2 : Gain  Gain=-SC_modul.R_esr
  Gain3 : Gain  Gain=1/n_sc_par
  Integrator : Integrator
  Product : Product  Inputs=3
  u_sc : Outport  InitialOutput=0  VectorParamsAs1DForOutWhenUnconnected=off
  "SoC_SC " : Outport  Port=2
  tag scope: SoC_SC=global, i_sc=global, i_sc_modul=global, u_sc=global, u_sc_modul=global
  wires:
  Integrator/1 -> Add/1
  Add/1 -> [u_sc_modul], Gain1/1
  i_sc/1 -> [i_sc], Gain3/1
  Gain/1 -> Integrator/1
  Constant/1 -> Add/2
  Gain1/1 -> Product/1, [u_sc], u_sc/1
  Gain2/1 -> Add/3
  Gain3/1 -> Gain2/1, Gain/1, [i_sc_modul]
  Constant1/1 -> Product/2
  Constant2/1 -> Product/3
  Product/1 -> "SoC_SC "/1, [SoC_SC]

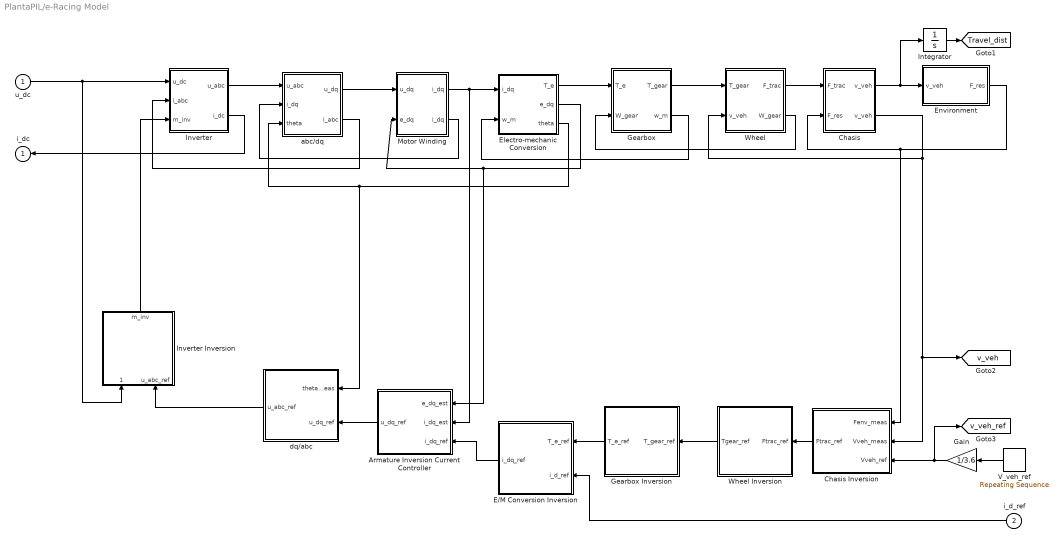
== system PlantaPIL/e-Racing Model ==
  u_dc : Inport
  i_d_ref : Inport  Port=2
  Armature Inversion Current Controller : Subsystem  AncestorBlock=simulink/SMC/Asservissement Correcteur IP
      mask Display: plot(0,0,100,100, [10,30,90,70,10,90],[90,10,10,90,90,10])
  Chasis : Subsystem  mask(CM){}
      mask Display: plot(0,0,100,100,[10,10,90,90,10],[90,10,10,90,90], [10,90],[10,90])
  "Chasis Inversion " : Subsystem  AncestorBlock=simulink/SMC/Asservissement Correcteur IP
      mask Display: plot(0,0,100,100, [10,30,90,70,10,90],[90,10,10,90,90,10])
  E/M Conversion Inversion : Subsystem  AncestorBlock=simulink/SMC/Inversion EC avec mesure
      mask Display: plot(0,0,100,100,[10,30,90,70,10],[90,10,10,90,90])
  Electro-mechanic Conversion : Subsystem
      mask Display: plot(0,0,100,100, 1.4*[50,57.68,60.77,63.08,64.97,66.58,68,69.26,70.4, 	71.42,72.36,78.28,80,78.28,72.36,71.42,70.4, 	69.26,68,66.58,64.97,63.08,60.77,57.68,50,42.32, 	39.23,36.92,35.03,33.42,32,30.74,29.6,28.58, 	27.64,21.72,20,21.72,27.64,28.58,29.6,30.74,32, 	33.42,35.03,36.92,39.23,42.32,50]-20, 1.4*[20,21,22,23,24,25,26,27,28,29,30,40,50,60,70,71,72, 	73,74,75,76,77,78,79,80,79,78,77,76,75,74,73,72, 	71,70,60,50,40,30,29,28,27,26,25,24,23,22,21,20]-20)
  Environment : Subsystem
      mask Display:
      | plot(0,0,100,100, 1.2*[50,57.68,60.77,63.08,64.97,66.58,68,69.26,70.4, 	71.42,72.36,78.28,80,78.28,72.36,71.42,70.4, 	69.26,68,66.58,64.97,63.08,60.77,57.68,50,42.32, 	39.23,36.92,35.03,33.42,32,30.74,29.6,28.58, 	27.64,21.72,20,21.72,27.64,28.58,29.6,30.74,32, 	33.42,35.03,36.92,39.23,42.32,50]-10, 1.2*[20,21,22,23,24,25,26,27,28,29,30,40,50,60,70,71,72, 	73,74,75,76,77,78,79,80,79,78,77,76,75,74,73,72, 	71,70,60,50,40,30,29,28,27,26,25,24,23,22,21,20]-10)
      | disp('Env.')
  Gain : Gain  Gain=1/3.6
  Gearbox : Subsystem
      mask Display: plot(0,0,100,100,[10,10,90,90,10],[90,10,10,90,90])
  Gearbox Inversion : Subsystem  AncestorBlock=simulink/SMC/Inversion EC avec mesure
      mask Display: plot(0,0,100,100,[10,30,90,70,10],[90,10,10,90,90])
  Integrator : Integrator
  Inverter : Subsystem
      mask Display: plot(0,0,100,100,[10,10,90,90,10],[90,10,10,90,90])
  Inverter Inversion : Subsystem  AncestorBlock=simulink/SMC/Inversion EC avec mesure
      mask Display: plot(0,0,100,100,[10,30,90,70,10],[90,10,10,90,90])
  Motor Winding : Subsystem  mask(CM){}
      mask Display: plot(0,0,100,100,[10,10,90,90,10],[90,10,10,90,90], [10,90],[10,90])
  V_veh_ref : simulink/Sources/Repeating Sequence  rep_seq_t=CYCL.time  rep_seq_y=CYCL.velocity
  Wheel : Subsystem
      mask Display: plot(0,0,100,100,[10,10,90,90,10],[90,10,10,90,90])
  "Wheel Inversion " : Subsystem  AncestorBlock=simulink/SMC/Inversion EC avec mesure
      mask Display: plot(0,0,100,100,[10,30,90,70,10],[90,10,10,90,90])
  abc/dq : Subsystem
      mask Display: plot(0,0,100,100,[10,10,90,90,10],[90,10,10,90,90])
  dq/abc : Subsystem  AncestorBlock=simulink/SMC/Inversion EC avec mesure
      mask Display: plot(0,0,100,100,[10,30,90,70,10],[90,10,10,90,90])
  i_dc : Outport  InitialOutput=0  VectorParamsAs1DForOutWhenUnconnected=off
  tag scope: Travel_dist=global, v_veh=global, v_veh_ref=global
  wires:
  Chasis/1(v_veh) -> Integrator/1, Environment/1(v_veh)
  "Wheel Inversion "/1(Tgear_ref) -> Gearbox Inversion/1(T_gear_ref)
  Gearbox/1(T_gear) -> Wheel/1(T_gear)
  Gearbox/2(w_m) -> Electro-mechanic Conversion/2(w_m)
  Environment/1(F_res) -> "Chasis Inversion "/1(Fenv_meas), Chasis/2(F_res)
  Electro-mechanic Conversion/3(theta) -> abc/dq/3(theta), dq/abc/1(theta_meas)
  dq/abc/1(u_abc_ref) -> Inverter Inversion/2(u_abc_ref)
  abc/dq/1(u_dq) -> Motor Winding/1(u_dq)
  Armature Inversion Current Controller/1(u_dq_ref) -> dq/abc/2(u_dq_ref)
  Inverter/2(i_dc) -> i_dc/1
  Gearbox Inversion/1(T_e_ref) -> E/M Conversion Inversion/1(T_e_ref)
  Chasis/2("v_veh  ") -> Wheel/2(v_veh), [v_veh], "Chasis Inversion "/2(Vveh_meas)
  u_dc/1 -> Inverter/1(u_dc), Inverter Inversion/1("u_dc_meas ")
  E/M Conversion Inversion/1(i_dq_ref) -> Armature Inversion Current Controller/3(i_dq_ref)
  Motor Winding/1(i_dq) -> Armature Inversion Current Controller/2(i_dq_est), Electro-mechanic Conversion/1(i_dq)
  Wheel/2(W_gear) -> Gearbox/2(W_gear)
  "Chasis Inversion "/1(Ftrac_ref) -> "Wheel Inversion "/1(Ftrac_ref)
  abc/dq/2(i_abc) -> Inverter/2(i_abc)
  Inverter Inversion/1(m_inv) -> Inverter/3(m_inv)
  Motor Winding/2("i_dq ") -> abc/dq/2(i_dq)
  Wheel/1(F_trac) -> Chasis/1(F_trac)
  Electro-mechanic Conversion/1(T_e) -> Gearbox/1(T_e)
  Electro-mechanic Conversion/2(e_dq) -> Armature Inversion Current Controller/1(e_dq_est), Motor Winding/2(e_dq)
  Inverter/1(u_abc) -> abc/dq/1(u_abc)
  Gain/1 -> [v_veh_ref], "Chasis Inversion "/3(Vveh_ref)
  Integrator/1 -> [Travel_dist]
  V_veh_ref/1 -> Gain/1
  i_d_ref/1 -> E/M Conversion Inversion/2(i_d_ref)

== system PlantaPIL/DC-bus Inversion/SC Limitation ==
  i_dc : Inport
  u_sc_meas : Inport  Port=2
  i_bat_ref_cal : Inport  Port=3
  Add : Sum  Inputs=+-
  Constant3 : Constant
  Divide : Product  Inputs=**
  Divide1 : Product  Inputs=**
  Limitation transition : Subsystem
  Sum : Sum
  i_bat_ref : Outport  VectorParamsAs1DForOutWhenUnconnected=off
  wires:
  Sum/1 -> i_bat_ref/1
  u_sc_meas/1 -> Limitation transition/3(u_sc_meas)
  Limitation transition/1(k_d) -> Add/2, Divide1/2
  Add/1 -> Divide/2
  Divide/1 -> Sum/2
  Divide1/1 -> Sum/1
  Constant3/1 -> Add/1
  i_dc/1 -> Divide1/1, Limitation transition/1(i_dc_meas)
  i_bat_ref_cal/1 -> Divide/1, Limitation transition/2(i_bat_ref_cal)

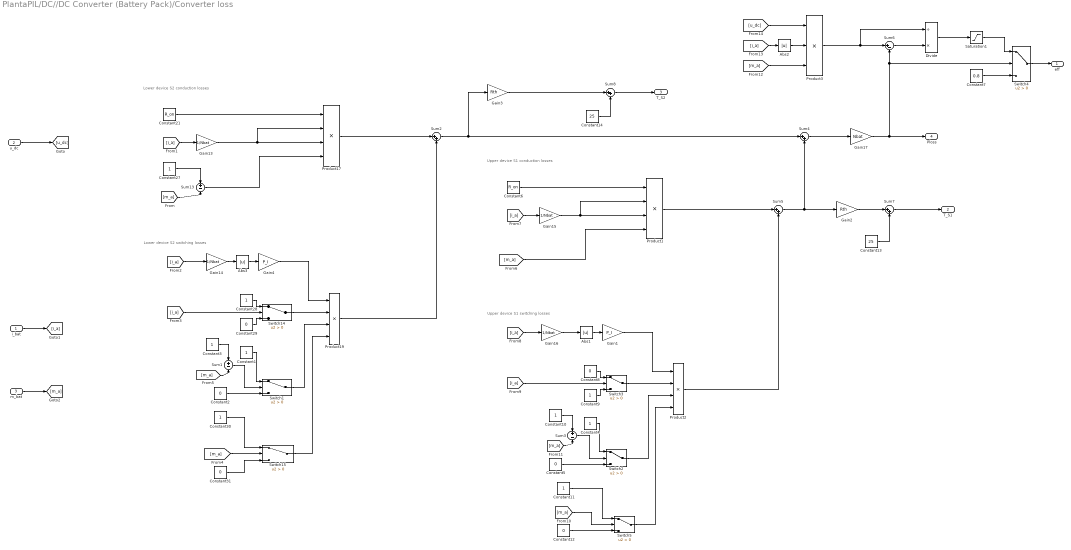
== system PlantaPIL/DC//DC Converter (Battery Pack)/Converter loss ==
  note: Lower device S2 conduction losses
  note: Lower device S2 switching losses
  note: Upper device S1 conduction losses
  note: Upper device S1 switching losses
  i_bat : Inport
  u_dc : Inport  Port=2
  m_bat : Inport  Port=3
  Abs1 : Abs  SaturateOnIntegerOverflow=off
  Abs2 : Abs  SaturateOnIntegerOverflow=off
  Abs3 : Abs  SaturateOnIntegerOverflow=off
  Constant{1,3..4,9..11,27..28,30} (9 alike) : Constant
  Constant{2,5,8,12,29,31} (6 alike) : Constant  Value=0
  Constant13 : Constant  Value=25
  Constant14 : Constant  Value=25
  Constant21 : Constant  Value=R_on
  Constant6 : Constant  Value=R_on
  Constant7 : Constant  Value=0.8
  Divide : Product  Inputs=/*
  Gain1 : Gain  Gain=P_I
  Gain{13..16} (4 alike) : Gain  Gain=1/Nbat
  Gain17 : Gain  Gain=Nbat
  Gain2 : Gain  Gain=Rth
  Gain3 : Gain  Gain=Rth
  Gain4 : Gain  Gain=P_I
  Product{1..2,17,19} (4 alike) : Product  Inputs=4
  Product3 : Product  Inputs=3
  Saturation1 : Saturate  UpperLimit=1  LowerLimit=0
  Sum1 : Sum  Inputs=+-
  Sum13 : Sum  Inputs=+-
  Sum{2,4..5,7..8} (5 alike) : Sum  Inputs=|++
  Sum3 : Sum  Inputs=+-
  Sum6 : Sum  Inputs=|+-
  Switch{1..5,14..15} (7 alike) : Switch  Criteria=u2 > Threshold  SaturateOnIntegerOverflow=off  InputSameDT=off
  eff : Outport
  T_S1 : Outport  Port=2
  T_S2 : Outport  Port=3
  Ploss : Outport  Port=4
  wires:
  m_bat/1 -> [m_a]
  Switch4/1 -> eff/1
  Constant7/1 -> Switch4/3
  Saturation1/1 -> Switch4/1
  Switch15/1 -> Product19/4
  Constant3/1 -> Sum1/1
  [m_a] -> Switch15/2
  [i_a] -> Gain14/1
  Constant27/1 -> Sum13/1
  [m_a] -> Sum13/2
  Switch14/1 -> Product19/2
  Gain4/1 -> Product19/1
  Constant28/1 -> Switch14/1
  Constant31/1 -> Switch15/3
  [m_a] -> Sum1/2
  Sum13/1 -> Product17/4
  Constant29/1 -> Switch14/3
  Abs3/1 -> Gain4/1
  Switch1/1 -> Product19/3
  [i_a] -> Switch14/2
  Constant2/1 -> Switch1/3
  Gain14/1 -> Abs3/1
  Product19/1 -> Sum2/2
  Product17/1 -> Sum2/1
  Constant30/1 -> Switch15/1
  Sum1/1 -> Switch1/2
  Constant1/1 -> Switch1/1
  [i_a] -> Gain13/1
  Gain13/1 -> Product17/2, Product17/3
  u_dc/1 -> [u_dc]
  i_bat/1 -> [i_a]
  [i_a] -> Gain16/1
  [m_a] -> Product1/4
  Constant9/1 -> Switch3/3
  Constant4/1 -> Switch2/1
  Constant6/1 -> Product1/1
  Constant10/1 -> Sum3/1
  [m_a] -> Sum3/2
  Switch3/1 -> Product2/2
  Switch2/1 -> Product2/3
  Gain1/1 -> Product2/1
  Constant11/1 -> Switch5/1
  Constant8/1 -> Switch3/1
  Sum3/1 -> Switch2/2
  [i_a] -> Gain15/1
  Constant5/1 -> Switch2/3
  Sum5/1 -> Gain2/1, Sum4/2
  [m_a] -> Switch5/2
  Product1/1 -> Sum5/1
  Gain15/1 -> Product1/2, Product1/3
  Product2/1 -> Sum5/2
  Constant12/1 -> Switch5/3
  Gain16/1 -> Abs1/1
  Abs1/1 -> Gain1/1
  [i_a] -> Switch3/2
  Switch5/1 -> Product2/4
  Sum4/1 -> Gain17/1
  Gain17/1 -> Ploss/1, Sum6/2, Switch4/2
  Sum2/1 -> Sum4/1, Gain3/1
  [i_a] -> Abs2/1
  [u_dc] -> Product3/1
  [m_a] -> Product3/3
  Product3/1 -> Divide/1, Sum6/1
  Abs2/1 -> Product3/2
  Sum6/1 -> Divide/2
  Divide/1 -> Saturation1/1
  Gain2/1 -> Sum7/1
  Sum7/1 -> T_S1/1
  Constant13/1 -> Sum7/2
  Gain3/1 -> Sum8/1
  Constant14/1 -> Sum8/2
  Sum8/1 -> T_S2/1
  Constant21/1 -> Product17/1

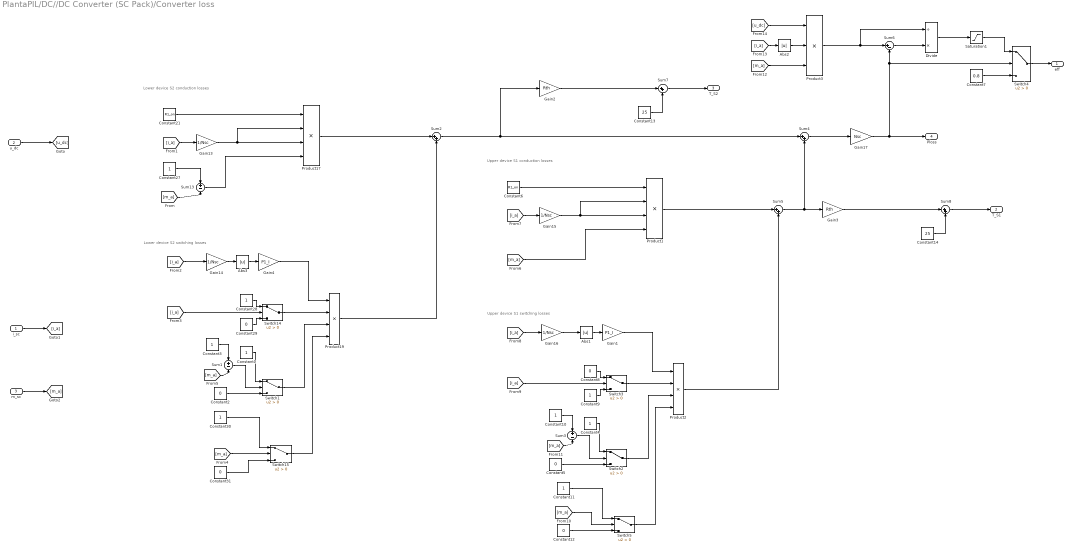
== system PlantaPIL/DC//DC Converter (SC Pack)/Converter loss ==
  note: Lower device S2 conduction losses
  note: Lower device S2 switching losses
  note: Upper device S1 conduction losses
  note: Upper device S1 switching losses
  i_sc : Inport
  u_dc : Inport  Port=2
  m_sc : Inport  Port=3
  Abs1 : Abs  SaturateOnIntegerOverflow=off
  Abs2 : Abs  SaturateOnIntegerOverflow=off
  Abs3 : Abs  SaturateOnIntegerOverflow=off
  Constant{1,3..4,9..11,27..28,30} (9 alike) : Constant
  Constant{2,5,8,12,29,31} (6 alike) : Constant  Value=0
  Constant13 : Constant  Value=25
  Constant14 : Constant  Value=25
  Constant21 : Constant  Value=R1_on
  Constant6 : Constant  Value=R1_on
  Constant7 : Constant  Value=0.8
  Divide : Product  Inputs=/*
  Gain1 : Gain  Gain=P1_I
  Gain{13..16} (4 alike) : Gain  Gain=1/Nsc
  Gain17 : Gain  Gain=Nsc
  Gain2 : Gain  Gain=Rth
  Gain3 : Gain  Gain=Rth
  Gain4 : Gain  Gain=P1_I
  Product{1..2,17,19} (4 alike) : Product  Inputs=4
  Product3 : Product  Inputs=3
  Saturation1 : Saturate  UpperLimit=1  LowerLimit=0
  Sum1 : Sum  Inputs=+-
  Sum13 : Sum  Inputs=+-
  Sum{2,4..5,7..8} (5 alike) : Sum  Inputs=|++
  Sum3 : Sum  Inputs=+-
  Sum6 : Sum  Inputs=|+-
  Switch{1..5,14..15} (7 alike) : Switch  Criteria=u2 > Threshold  SaturateOnIntegerOverflow=off  InputSameDT=off
  eff : Outport
  T_S1 : Outport  Port=2
  T_S2 : Outport  Port=3
  Ploss : Outport  Port=4
  wires:
  m_sc/1 -> [m_a]
  Switch4/1 -> eff/1
  Constant7/1 -> Switch4/3
  Saturation1/1 -> Switch4/1
  Switch15/1 -> Product19/4
  Constant3/1 -> Sum1/1
  [m_a] -> Switch15/2
  [i_a] -> Gain14/1
  Constant27/1 -> Sum13/1
  [m_a] -> Sum13/2
  Switch14/1 -> Product19/2
  Gain4/1 -> Product19/1
  Constant28/1 -> Switch14/1
  Constant31/1 -> Switch15/3
  [m_a] -> Sum1/2
  Sum13/1 -> Product17/4
  Constant29/1 -> Switch14/3
  Abs3/1 -> Gain4/1
  Switch1/1 -> Product19/3
  [i_a] -> Switch14/2
  Constant2/1 -> Switch1/3
  Gain14/1 -> Abs3/1
  Product19/1 -> Sum2/2
  Product17/1 -> Sum2/1
  Constant30/1 -> Switch15/1
  Sum1/1 -> Switch1/2
  Constant1/1 -> Switch1/1
  [i_a] -> Gain13/1
  Gain13/1 -> Product17/2, Product17/3
  Constant21/1 -> Product17/1
  u_dc/1 -> [u_dc]
  i_sc/1 -> [i_a]
  [i_a] -> Gain16/1
  [m_a] -> Product1/4
  Constant9/1 -> Switch3/3
  Constant4/1 -> Switch2/1
  Constant6/1 -> Product1/1
  Constant10/1 -> Sum3/1
  [m_a] -> Sum3/2
  Switch3/1 -> Product2/2
  Switch2/1 -> Product2/3
  Gain1/1 -> Product2/1
  Constant11/1 -> Switch5/1
  Constant8/1 -> Switch3/1
  Sum3/1 -> Switch2/2
  [i_a] -> Gain15/1
  Constant5/1 -> Switch2/3
  Sum5/1 -> Gain3/1, Sum4/2
  [m_a] -> Switch5/2
  Product1/1 -> Sum5/1
  Gain15/1 -> Product1/2, Product1/3
  Product2/1 -> Sum5/2
  Constant12/1 -> Switch5/3
  Gain16/1 -> Abs1/1
  Abs1/1 -> Gain1/1
  [i_a] -> Switch3/2
  Switch5/1 -> Product2/4
  Sum4/1 -> Gain17/1
  Gain17/1 -> Ploss/1, Sum6/2, Switch4/2
  Sum2/1 -> Gain2/1, Sum4/1
  [i_a] -> Abs2/1
  [u_dc] -> Product3/1
  [m_a] -> Product3/3
  Product3/1 -> Divide/1, Sum6/1
  Abs2/1 -> Product3/2
  Sum6/1 -> Divide/2
  Divide/1 -> Saturation1/1
  Constant14/1 -> Sum8/2
  Sum8/1 -> T_S1/1
  Gain3/1 -> Sum8/1
  Gain2/1 -> Sum7/1
  Sum7/1 -> T_S2/1
  Constant13/1 -> Sum7/2

== system PlantaPIL/Proposed Strategy/Variables controlador ==
  Constant : Constant  Value=10^-4
  Product : Product  Inputs=3
  Sum : Sum  Inputs=+-
  SoC_Bat : Outport
  SoC_SC : Outport  Port=2
  Potencia_Req : Outport  Port=3
  Velocidad_w : Outport  Port=4
  ErrorVelocidad : Outport  Port=5
  wires:
  [w_m] -> Velocidad_w/1
  [u_dc] -> Product/1
  [i_dc] -> Product/2
  Constant/1 -> Product/3
  [v_veh_ref] -> Sum/1
  [v_veh] -> Sum/2
  [Bat_soc] -> SoC_Bat/1
  [SoC_SC] -> SoC_SC/1
  Product/1 -> Potencia_Req/1
  Sum/1 -> ErrorVelocidad/1

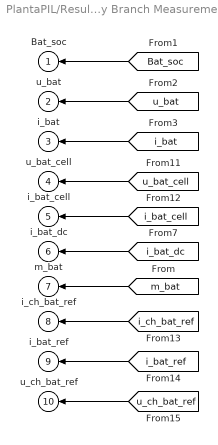
== system PlantaPIL/Results Collecting for Scoring/Battery Branch Measurement ==
  Bat_soc : Outport  VectorParamsAs1DForOutWhenUnconnected=off
  u_bat : Outport  Port=2  VectorParamsAs1DForOutWhenUnconnected=off
  i_bat : Outport  Port=3  VectorParamsAs1DForOutWhenUnconnected=off
  u_bat_cell : Outport  Port=4  VectorParamsAs1DForOutWhenUnconnected=off
  i_bat_cell : Outport  Port=5  VectorParamsAs1DForOutWhenUnconnected=off
  i_bat_dc : Outport  Port=6  VectorParamsAs1DForOutWhenUnconnected=off
  m_bat : Outport  Port=7  VectorParamsAs1DForOutWhenUnconnected=off
  i_ch_bat_ref : Outport  Port=8  VectorParamsAs1DForOutWhenUnconnected=off
  i_bat_ref : Outport  Port=9  VectorParamsAs1DForOutWhenUnconnected=off
  u_ch_bat_ref : Outport  Port=10  VectorParamsAs1DForOutWhenUnconnected=off
  wires:
  [Bat_soc] -> Bat_soc/1
  [u_bat] -> u_bat/1
  [i_bat] -> i_bat/1
  [u_bat_cell] -> u_bat_cell/1
  [i_bat_cell] -> i_bat_cell/1
  [i_bat_dc] -> i_bat_dc/1
  [m_bat] -> m_bat/1
  [i_ch_bat_ref] -> i_ch_bat_ref/1
  [i_bat_ref] -> i_bat_ref/1
  [u_ch_bat_ref] -> u_ch_bat_ref/1

== system PlantaPIL/Results Collecting for Scoring/Losses and Temperatures ==
  Ploss_bat : Outport  VectorParamsAs1DForOutWhenUnconnected=off
  Ploss_sc : Outport  Port=2  VectorParamsAs1DForOutWhenUnconnected=off
  Ploss_inv : Outport  Port=3  VectorParamsAs1DForOutWhenUnconnected=off
  Ploss_em : Outport  Port=4  VectorParamsAs1DForOutWhenUnconnected=off
  Ts1_bat : Outport  Port=5  VectorParamsAs1DForOutWhenUnconnected=off
  Ts2_bat : Outport  Port=6  VectorParamsAs1DForOutWhenUnconnected=off
  Ts1_sc : Outport  Port=7  VectorParamsAs1DForOutWhenUnconnected=off
  Ts2_sc : Outport  Port=8  VectorParamsAs1DForOutWhenUnconnected=off
  Ts1_inv : Outport  Port=9  VectorParamsAs1DForOutWhenUnconnected=off
  Ts2_inv : Outport  Port=10  VectorParamsAs1DForOutWhenUnconnected=off
  wires:
  [Ploss_bat] -> Ploss_bat/1
  [Ploss_sc] -> Ploss_sc/1
  [Ploss_em] -> Ploss_em/1
  [Ploss_inv] -> Ploss_inv/1
  [Ts2_sc] -> Ts2_sc/1
  [Ts1_sc] -> Ts1_sc/1
  [Ts2_bat] -> Ts2_bat/1
  [Ts1_bat] -> Ts1_bat/1
  [Ts1_inv] -> Ts1_inv/1
  [Ts2_inv] -> Ts2_inv/1

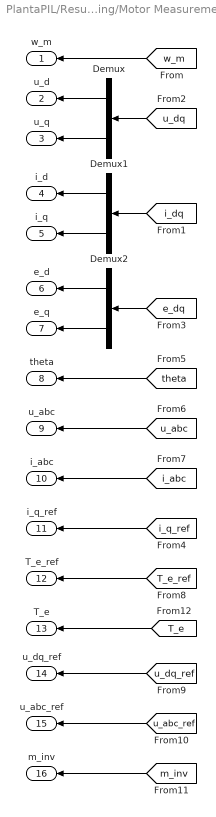
== system PlantaPIL/Results Collecting for Scoring/Motor Measurement ==
  Demux : Demux  Outputs=2
  Demux1 : Demux  Outputs=2
  Demux2 : Demux  Outputs=2
  w_m : Outport
  u_d : Outport  Port=2
  u_q : Outport  Port=3
  i_d : Outport  Port=4
  i_q : Outport  Port=5
  e_d : Outport  Port=6
  e_q : Outport  Port=7
  theta : Outport  Port=8
  u_abc : Outport  Port=9
  i_abc : Outport  Port=10
  i_q_ref : Outport  Port=11
  T_e_ref : Outport  Port=12
  T_e : Outport  Port=13
  u_dq_ref : Outport  Port=14
  u_abc_ref : Outport  Port=15
  m_inv : Outport  Port=16
  wires:
  [u_dq] -> Demux/1
  [i_dq] -> Demux1/1
  [w_m] -> w_m/1
  Demux/1 -> u_d/1
  Demux/2 -> u_q/1
  Demux1/1 -> i_d/1
  Demux1/2 -> i_q/1
  [e_dq] -> Demux2/1
  Demux2/1 -> e_d/1
  Demux2/2 -> e_q/1
  [theta] -> theta/1
  [u_abc] -> u_abc/1
  [i_abc] -> i_abc/1
  [i_q_ref] -> i_q_ref/1
  [T_e_ref] -> T_e_ref/1
  [u_dq_ref] -> u_dq_ref/1
  [u_abc_ref] -> u_abc_ref/1
  [m_inv] -> m_inv/1
  [T_e] -> T_e/1
